simulink model "TP1_simulink"  (R2023b)
settings: Solver=VariableStepAuto  StartTime=0.0  StopTime=60  RelTol=1e-3
undefined symbols (not defined in the file): A, A_tau, B, E, f_tau, t_p
libraries: slpidlib x1
settings Model: Creator=robot  LastModifiedBy=robot

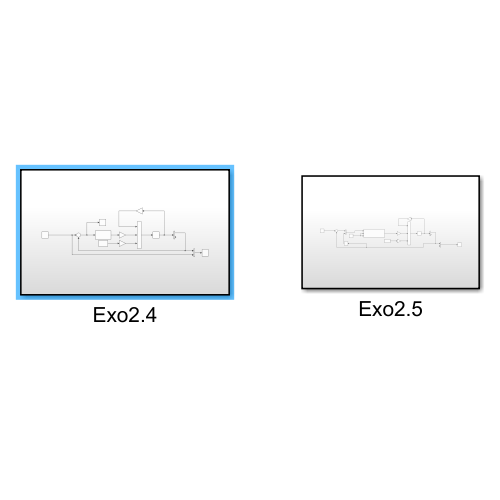
[thumbnail: Simulink's stored preview of the top-level diagram]
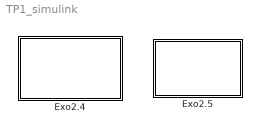
== system TP1_simulink ==
  Exo2.4 : Subsystem
  Exo2.5 : Subsystem

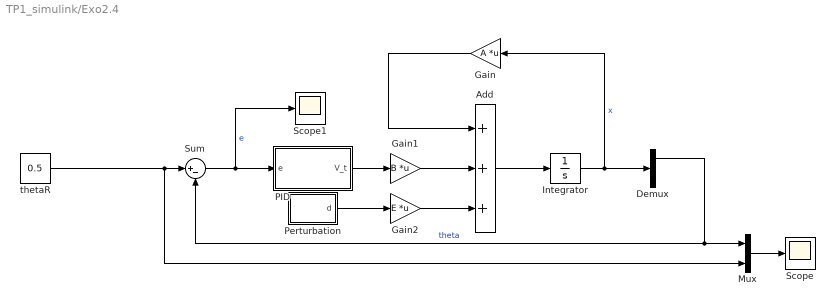
== system TP1_simulink/Exo2.4 ==
  Add : Sum  Inputs=+++
  Demux : Demux  Outputs=2
  Gain : Gain  Gain=A  Multiplication=Matrix(K*u)
  Gain1 : Gain  Gain=B  Multiplication=Matrix(K*u)
  Gain2 : Gain  Gain=E  Multiplication=Matrix(K*u)
  Integrator : Integrator
  Mux : Mux  Inputs=2
  PID : Subsystem
  Perturbation : Subsystem
  Scope : Scope
  Scope1 : Scope
  Sum : Sum  Inputs=|+-
  thetaR : Constant  Value=0.5
  wires:
  thetaR/1 -> Mux/2, Sum/1
  Gain2/1 -> Add/3
  Sum/1 -> Scope1/1, PID/1(e)  "e"
  Demux/1 -> Sum/2, Mux/1  "theta"
  PID/1(V_t) -> Gain1/1
  Mux/1 -> Scope/1
  Integrator/1 -> Demux/1, Gain/1  "x"
  Add/1 -> Integrator/1
  Gain1/1 -> Add/2
  Gain/1 -> Add/1
  Perturbation/1(d) -> Gain2/1

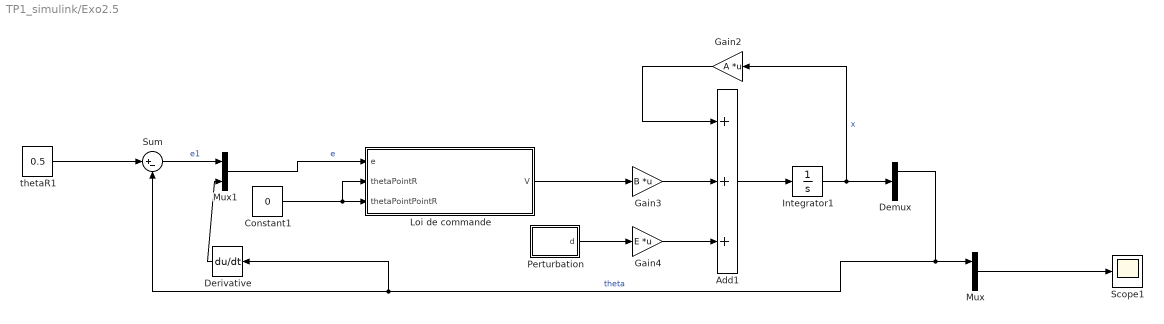
== system TP1_simulink/Exo2.5 ==
  Add1 : Sum  Inputs=+++
  Constant1 : Constant  Value=0
  Demux : Demux  Outputs=2
  Derivative : Derivative
  Gain2 : Gain  Gain=A  Multiplication=Matrix(K*u)
  Gain3 : Gain  Gain=B  Multiplication=Matrix(K*u)
  Gain4 : Gain  Gain=E  Multiplication=Matrix(K*u)
  Integrator1 : Integrator
  Loi de commande : MATLAB Function  TreatAsAtomicUnit=on
  Mux : Mux  Inputs=2
  Mux1 : Mux  Inputs=2
  Perturbation : Subsystem
  Scope1 : Scope
  Sum : Sum  Inputs=|+-
  thetaR1 : Constant  Value=0.5
  wires:
  Perturbation/1(d) -> Gain4/1
  Integrator1/1 -> Demux/1, Gain2/1  "x"
  Gain2/1 -> Add1/1
  Mux/1 -> Scope1/1
  Gain3/1 -> Add1/2
  Gain4/1 -> Add1/3
  Add1/1 -> Integrator1/1
  thetaR1/1 -> Sum/1
  Demux/1 -> Sum/2, Derivative/1, Mux/1  "theta"
  Constant1/1 -> Loi de commande/3(thetaPointPointR), Loi de commande/2(thetaPointR)
  Loi de commande/1(V) -> Gain3/1
  Sum/1 -> Mux1/1  "e1"
  Mux1/1 -> Loi de commande/1(e)  "e"
  Derivative/1 -> Mux1/2

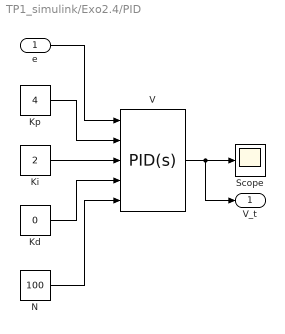
== system TP1_simulink/Exo2.4/PID ==
  e : Inport
  Kd : Constant  Value=0
  Ki : Constant  Value=2
  Kp : Constant  Value=4
  N : Constant  Value=100
  Scope : Scope
  V : slpidlib/PID Controller  Controller=PID  Form=Parallel  TimeDomain=Continuous-time  UseExternalTs=off  SampleTime=-1  IntegratorMethod=Forward Euler  FilterMethod=Forward Euler  ControllerParametersSource=external  P=1  I=1  UseKiTs=off  D=0  N=100  UseFilter=on  TunerSelectOption=Transfer Function Based (PID Tuner App)  InitialConditionSource=internal  InitialConditionForIntegrator=0  InitialConditionForFilter=0  DifferentiatorICPrevScaledInput=0  ExternalReset=none  TrackingMode=off  Kt=1  LimitOutput=on  SatLimitsSource=internal  UpperSaturationLimit=12  LowerSaturationLimit=-12  LinearizeAsGain=on  AntiWindupMode=none  Kb=1  LimitIntegrator=off  UpperIntegratorSaturationLimit=inf  LowerIntegratorSaturationLimit=-inf  POutMin=[]  POutMax=[]  IOutMin=[]  IOutMax=[]  DOutMin=[]  DOutMax=[]  NOutMin=[]  NOutMax=[]  SumOutMin=[]  SumOutMax=[]  SaturationOutMin=[]  SaturationOutMax=[]  PParamMin=[]  PParamMax=[]  IParamMin=[]  IParamMax=[]  DParamMin=[]  DParamMax=[]  NParamMin=[]  NParamMax=[]  KbParamMin=[]  KbParamMax=[]  KtParamMin=[]  KtParamMax=[]  KbOutMin=[]  KbOutMax=[]  KtOutMin=[]  KtOutMax=[]  IntegratorOutMin=[]  IntegratorOutMax=[]  FilterOutMin=[]  FilterOutMax=[]  SumI1OutMin=[]  SumI1OutMax=[]  SumI2OutMin=[]  SumI2OutMax=[]  SumI3OutMin=[]  SumI3OutMax=[]  SumI4OutMin=[]  SumI4OutMax=[]  SumDOutMin=[]  SumDOutMax=[]  DifferentiatorOutMin=[]  DifferentiatorOutMax=[]  FilterDiffOutCoefMin=[]  FilterDiffOutCoefMax=[]  ReciprocalOutMin=[]  ReciprocalOutMax=[]  SumDenOutMin=[]  SumDenOutMax=[]  SumNumOutMin=[]  SumNumOutMax=[]  DivideOutMin=[]  DivideOutMax=[]  UdiffTsProdOutMin=[]  UdiffTsProdOutMax=[]  NTsProdOutMin=[]  NTsProdOutMax=[]  UintegralTsProdOutMin=[]  UintegralTsProdOutMax=[]  UngainTsProdOutMin=[]  UngainTsProdOutMax=[]  ClampingZeroOutDataTypeStr=Inherit: Inherit via back propagation  ClampingZeroOutMin=[]  ClampingZeroOutMax=[]  FilterDenConstantOutDataTypeStr=Inherit: Inherit via back propagation  FilterDenConstantOutMin=[]  FilterDenConstantOutMax=[]  PCopyOutDataTypeStr=Inherit: Inherit via back propagation  PCopyOutMin=[]  PCopyOutMax=[]  NCopyOutDataTypeStr=Inherit: Inherit via back propagation  NCopyOutMin=[]  NCopyOutMax=[]  IntegratorContinuousStateAttributes=''  IntegratorStateMustResolveToSignalObject=off  IntegratorRTWStateStorageClass=Auto  FilterContinuousStateAttributes=''  FilterStateMustResolveToSignalObject=off  FilterRTWStateStorageClass=Auto  ParallelPVariant=ExternalParameters  IdealPVariant=Disabled  IVariant=ExternalParameters  DVariant=ExternalParameters  IntegratorVariant=Continuous  SatVariant=Enabled  AWVariant=Passthrough  PCopyVariant=Disabled  TRVariant=Disabled  FdbkBlocksVariant=Forward  IdealPFdbkVariant=Disabled  SatFdbkVariant=Disabled  DerivativeFilterVariant=ContFilter  NVariant=ExternalParameters  NCopyVariant=Disabled  FilterICVariant=InternalICsFilter  IntegratorICVariant=InternalICs  ExternalResetVariant=Disabled  TRSumVariant=Passthrough  SumFdbkVariant=Disabled  SumVariant=Sum_PID  TsampFilterVariant=InternalTs  TsampNgainVariant=Passthrough  TsampIntegralVariant=Disabled_SignalSpec  ExternalSaturationOutDataTypeStr=Inherit: Same as second input
  V_t : Outport
  wires:
  Ki/1 -> V/3
  e/1 -> V/1
  Kp/1 -> V/2
  Kd/1 -> V/4
  N/1 -> V/5
  V/1 -> Scope/1, V_t/1

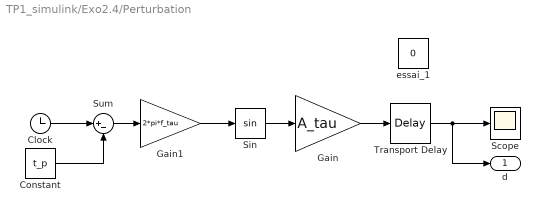
== system TP1_simulink/Exo2.4/Perturbation ==
  Clock : Clock
  Constant : Constant  Value=t_p
  Gain : Gain  Gain=A_tau
  Gain1 : Gain  Gain=2*pi*f_tau
  Scope : Scope
  Sin : Trigonometry
  Sum : Sum  Inputs=|+-
  Transport Delay : TransportDelay  DelayTime=3
  essai_1 : Constant  Value=0
  d : Outport
  wires:
  Clock/1 -> Sum/1
  Constant/1 -> Sum/2
  Sum/1 -> Gain1/1
  Gain1/1 -> Sin/1
  Sin/1 -> Gain/1
  Gain/1 -> Transport Delay/1
  Transport Delay/1 -> d/1, Scope/1

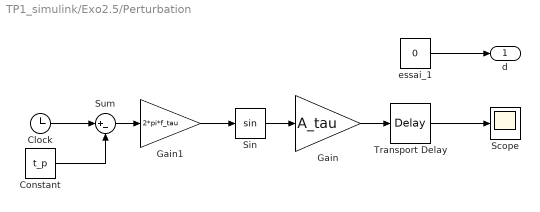
== system TP1_simulink/Exo2.5/Perturbation ==
  Clock : Clock
  Constant : Constant  Value=t_p
  Gain : Gain  Gain=A_tau
  Gain1 : Gain  Gain=2*pi*f_tau
  Scope : Scope
  Sin : Trigonometry
  Sum : Sum  Inputs=|+-
  Transport Delay : TransportDelay  DelayTime=3
  essai_1 : Constant  Value=0
  d : Outport
  wires:
  Clock/1 -> Sum/1
  Constant/1 -> Sum/2
  Sum/1 -> Gain1/1
  Gain1/1 -> Sin/1
  Sin/1 -> Gain/1
  Gain/1 -> Transport Delay/1
  Transport Delay/1 -> Scope/1
  essai_1/1 -> d/1

== matlab function TP1_simulink/Exo2.5/Loi de commande ==
  data: e input; V output; thetaPointR input; thetaPointPointR input
function V = fcn(e, thetaPointR, thetaPointPointR)
a_1 = 89.6304;
a_0 = 23.4652;

K = [21.0000  -79.6304];


V = (1/a_0).*(-K*e + a_1*thetaPointR + thetaPointPointR);
